simulink model "pid_LINEAR"  (R2022a)
settings: Solver=VariableStepAuto  StartTime=0.0  StopTime=200  RelTol=1e-3
settings Model: Creator=MY PC  LastModifiedBy=amogh
settings SolverCC: AlgebraicLoopSolver=TrustRegion
settings DebuggingCC: UnconnectedInputMsg=warning  UnconnectedOutputMsg=warning  UnconnectedLineMsg=warning  SFMachineParentedDataDiag=warning
settings RTWCC: DLArmComputeVersion=19.05

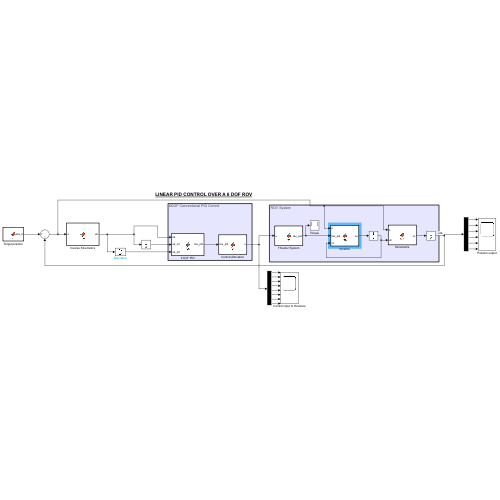
[thumbnail: Simulink's stored preview of the top-level diagram]
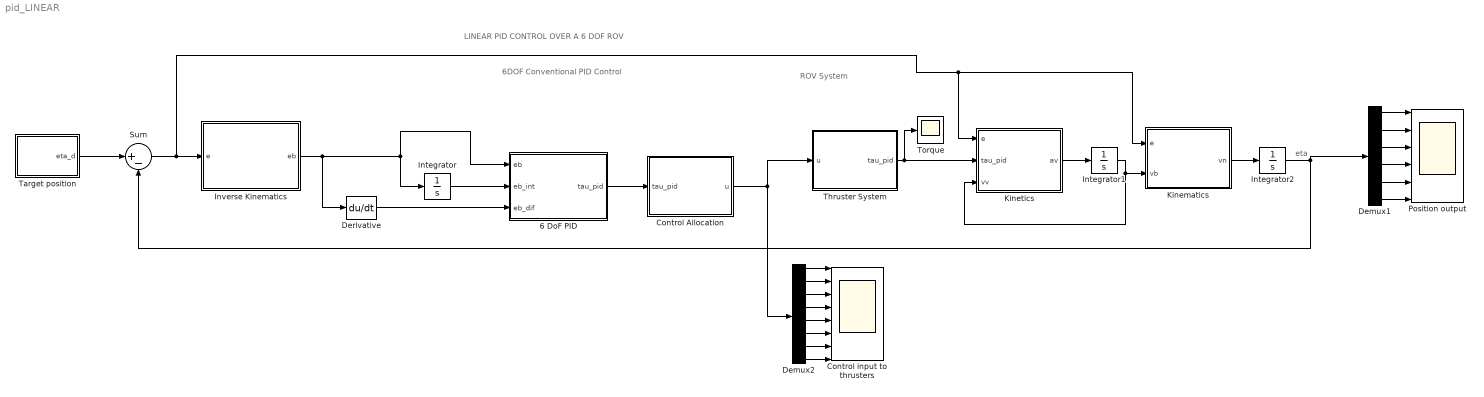
== system pid_LINEAR ==
  note: eta
  note: ROV System
  note: 6DOF Conventional PID Control
  note: LINEAR PID CONTROL OVER A 6 DOF ROV
  6 DoF PID : MATLAB Function  TreatAsAtomicUnit=on
  Control Allocation : MATLAB Function  TreatAsAtomicUnit=on
  Control input to thrusters : Scope  NumInputPorts=8
  Demux1 : Demux  Outputs=6
  Demux2 : Demux  Outputs=8
  Derivative : Derivative
  Integrator : Integrator  InitialCondition=[0;0;0;0;0;0]
  Integrator1 : Integrator  InitialCondition=[0;0;0;0;0;0]
  Integrator2 : Integrator  InitialCondition=[0;0;0;0;0;0]  ContinuousStateAttributes='eta'
  Inverse Kinematics : MATLAB Function  TreatAsAtomicUnit=on
  Kinematics : MATLAB Function  TreatAsAtomicUnit=on
  Kinetics : MATLAB Function  TreatAsAtomicUnit=on
  Position output : Scope  NumInputPorts=6
  Sum : Sum  Inputs=|+-
  Target position : MATLAB Function  TreatAsAtomicUnit=on
  Thruster System : MATLAB Function  TreatAsAtomicUnit=on
  Torque : Scope
  wires:
  Target position/1(eta_d) -> Sum/1
  Integrator2/1 -> Demux1/1, Sum/2
  Demux1/4 -> Position output/4
  Demux1/3 -> Position output/3
  Demux1/1 -> Position output/1
  Demux1/6 -> Position output/6
  Demux1/5 -> Position output/5
  Demux1/2 -> Position output/2
  Demux2/1 -> Control input to thrusters/1
  Demux2/2 -> Control input to thrusters/2
  Demux2/3 -> Control input to thrusters/3
  Demux2/4 -> Control input to thrusters/4
  Demux2/5 -> Control input to thrusters/5
  Demux2/6 -> Control input to thrusters/6
  Demux2/7 -> Control input to thrusters/7
  Demux2/8 -> Control input to thrusters/8
  Inverse Kinematics/1(eb) -> Integrator/1, 6 DoF PID/1(eb), Derivative/1
  Derivative/1 -> 6 DoF PID/3(eb_dif)
  Integrator/1 -> 6 DoF PID/2(eb_int)
  6 DoF PID/1(tau_pid) -> Control Allocation/1(tau_pid)
  Sum/1 -> Kinetics/1(e), Kinematics/1(e), Inverse Kinematics/1(e)
  Control Allocation/1(u) -> Thruster System/1(u), Demux2/1
  Thruster System/1(tau_pid) -> Torque/1, Kinetics/2(tau_pid)
  Integrator1/1 -> Kinetics/3(vv), Kinematics/2(vb)
  Kinetics/1(av) -> Integrator1/1
  Kinematics/1(vn) -> Integrator2/1

== matlab function pid_LINEAR/Target position ==
  data: eta_d output
function eta_d = fcn()

eta_d = [3;4;1;1.57;0;0];

== matlab function pid_LINEAR/Inverse Kinematics ==
  data: e input; eb output
function eb = fcn(e)

phi=e(4);
theta=e(5);
psi=e(6);
R=[cos(psi)*cos(theta),-sin(psi)*cos(phi)+cos(psi)*sin(theta)*sin(phi),sin(psi)*sin(phi)+cos(psi)*cos(phi)*sin(theta);
    sin(psi)*cos(theta),cos(psi)*cos(phi)+sin(psi)*sin(theta)*sin(phi),-cos(psi)*sin(phi)+sin(theta)*sin(psi)*cos(phi);
    -sin(theta),cos(theta)*sin(phi),cos(theta)*cos(phi)];

T=[1,sin(phi)*tan(theta),cos(phi)*tan(theta);
    0,cos(phi),-sin(phi);
    0,sin(phi)/cos(theta),cos(phi)/cos(theta)];

J=[R,zeros(3,3);zeros(3,3),T];

eb = transpose(J)*e;

== matlab function pid_LINEAR/6 DoF PID ==
  data: eb input; tau_pid output; eb_int input; eb_dif input
function tau_pid = fcn(eb,eb_int,eb_dif)

kp = [3;3;3;4;4;2];
ki = [0.2;0.2;0.2;0.3;0.3;0.1];
kd = [2.5;2.5;0.5;0.5;1;0.5];

tau_pid = kp.*eb + ki.*eb_int + kd.*eb_dif;

== matlab function pid_LINEAR/Control Allocation ==
  data: tau_pid input; u output
function u = fcn(tau_pid)

K = diag([40, 40, 40, 40, 40, 40, 40, 40]);

T = [0.707,0.707, -0.707, -0.707, 0, 0, 0, 0; 
    -0.707, 0.707, -0.707, 0.707, 0, 0, 0, 0;
    0, 0, 0, 0, -1, 1, 1, -1;
    0.06, -0.06, 0.06, -0.06, -0.218, -0.218, 0.218, 0.218;
    0.06, -0.06, 0.06, -0.06, 0.12, -0.12, 0.12, -0.12;
    -0.1888, 0.1888, 0.1888, -0.1888, 0, 0, 0, 0];
T_tran = transpose(T);
T_inv = T_tran*(inv(T*T_tran));
K_inv = inv(K);
u = (K_inv*T_inv)*tau_pid;

== matlab function pid_LINEAR/Thruster System ==
  data: u input; tau_pid output
function tau_pid = fcn(u)

K = diag([40, 40, 40, 40, 40, 40, 40, 40]);

T = [0.707,0.707, -0.707, -0.707, 0, 0, 0, 0; 
    -0.707, 0.707, -0.707, 0.707, 0, 0, 0, 0;
    0, 0, 0, 0, -1, 1, 1, -1;
    0.06, -0.06, 0.06, -0.06, -0.218, -0.218, 0.218, 0.218;
    0.06, -0.06, 0.06, -0.06, 0.12, -0.12, 0.12, -0.12;
    -0.1888, 0.1888, 0.1888, -0.1888, 0, 0, 0, 0];
tau_pid = (T*K)*u;

== matlab function pid_LINEAR/Kinetics ==
  data: e input; tau_pid input; av output; vv input
function av = fcn(e,tau_pid,vv)

m = 11.5;
g = 9.81;
zg = 0.02;
Ix = 0.16;
Iy = 0.16;
Iz = 0.16;
Xu_dot = -5.5;
Yv_dot = -12.7;
Zw_dot = -14.57;
Kp_dot = -0.12;
Mq_dot = -0.12;
Nr_dot = -0.12;
W = 112.8; % = m*g
B = 117.8; % = net buoyancy + W
phi=e(4);
theta=e(5);
u = vv(1);
v = vv(1);
w = vv(2);
p=vv(4);
q=vv(5);
r=vv(6);
MRB=[m,0,0,0,m*zg,0;
    0,m,0,-m*zg,0,0;
    0,0,m,0,0,0;
    0,-m*zg,0,Ix,0,0;
    m*zg,0,0,0,Iy,0;
    0,0,0,0,0,Iz
    ];
MA = (-1).*[Xu_dot,0,0,0,0,0;
          0,Yv_dot,0,0,0,0;
          0,0,Zw_dot,0,0,0;
          0,0,0,Kp_dot,0,0;
          0,0,0,0,Mq_dot,0;
          0,0,0,0,0,Nr_dot];
M = MRB+MA;
%vc = [0.1;0.1;0;0;0;0];
CRB = [0,0,0,0,m*w,0;
    0,0,0,-m*w,0,0;
    0,0,0,m*v,-m*u,0;
    0,m*w,-m*v,0,Iz*r,-Iy*q;
    -m*w,0,-m*u,-Iz*r,0,Ix*p;
    m*v,-m*u,0,Iy*q,-Ix*p,0];
CA = [0,0,0,0,Zw_dot*w,0;
    0,0,0,-1*Zw_dot*w,0,-1*Xu_dot*u;
    0,0,0,-1*Yv_dot*v,Xu_dot*u,0;
    0,-1*Zw_dot*w,Yv_dot*v,0,-1*Nr_dot*r,Mq_dot*q;
    Zw_dot*w,0,-1*Xu_dot*u,Nr_dot*r,0,-1*Kp_dot*p;
    -1*Yv_dot*v,Xu_dot*u,0,-1*Mq_dot*q,Kp_dot*p,0];
D=diag([4.03+18.18*abs(u),6.22+21.66*abs(v),5.18+36.99*abs(w),0.07+1.55*abs(p),0.07+1.55*abs(q),0.07+1.55*abs(r)]);
G=[(W-B)*sin(theta);-(W-B)*cos(theta)*sin(phi);-(W-B)*cos(theta)*cos(phi);zg*W*cos(theta)*sin(phi);zg*W*sin(theta);0];

vw = vv;

av = inv(M)*(tau_pid-G-((D+CA)*vw)-(CRB*vv));

== matlab function pid_LINEAR/Kinematics ==
  data: e input; vb input; vn output
function vn = fcn(e,vb)

phi=e(4);
theta=e(5);
psi=e(6);
R=[cos(psi)*cos(theta),-sin(psi)*cos(phi)+cos(psi)*sin(theta)*sin(phi),sin(psi)*sin(phi)+cos(psi)*cos(phi)*sin(theta);
   sin(psi)*cos(theta),cos(psi)*cos(phi)+sin(psi)*sin(theta)*sin(phi),-cos(psi)*sin(phi)+sin(theta)*sin(psi)*cos(phi);
   -sin(theta),cos(theta)*sin(phi),cos(theta)*cos(phi)];
T=[1,sin(phi)*tan(theta),cos(phi)*tan(theta);
    0,cos(phi),-sin(phi);
    0,sin(phi)/cos(theta),cos(phi)/cos(theta)];

J=[R,zeros(3,3);zeros(3,3),T];

vn=J*vb;
